simulink model "regulator_sistem_oscilant"  (R2023b)
settings: Solver=VariableStepAuto  StartTime=0.0  StopTime=100  MaxStep=1e-3  RelTol=1e-3
values from neighbouring files (symbols this model uses):
  den = [T 1]    [sns_proiect_Ceoca_Ovidiu.m]
  num = [1]    [sns_proiect_Ceoca_Ovidiu.m]
undefined symbols (not defined in the file or in its folder): Kp_ZN, Ti_ZN
settings Model: Creator=ovidiuceoca  LastModifiedBy=ovidiuceoca

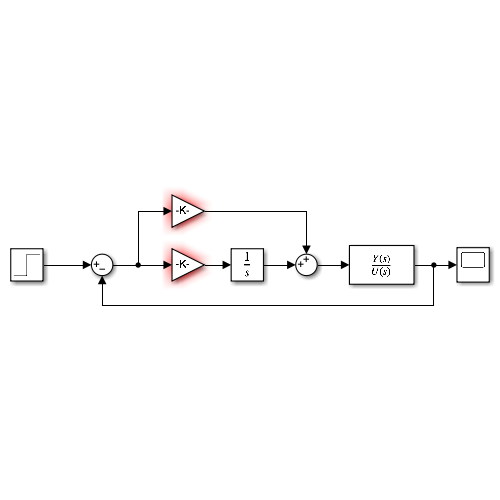
[thumbnail: Simulink's stored preview of the top-level diagram]
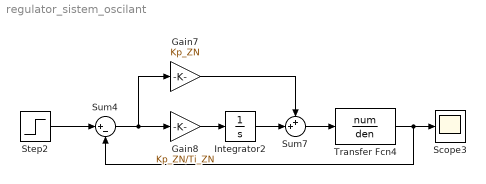
== system regulator_sistem_oscilant ==
  Gain7 : Gain  Gain=Kp_ZN
  Gain8 : Gain  Gain=Kp_ZN/Ti_ZN
  Integrator2 : Integrator
  Scope3 : Scope
  Step2 : Step  Time=0  SampleTime=0
  Sum4 : Sum  Inputs=|+-
  Sum7 : Sum  Inputs=++|
  Transfer Fcn4 : TransferFcn  Numerator=num  Denominator=den
  wires:
  Step2/1 -> Sum4/1
  Sum7/1 -> Transfer Fcn4/1
  Gain8/1 -> Integrator2/1
  Sum4/1 -> Gain7/1, Gain8/1
  Transfer Fcn4/1 -> Sum4/2, Scope3/1
  Gain7/1 -> Sum7/1
  Integrator2/1 -> Sum7/2
